simulink model "main_simulation"  (R2021a)
settings: Solver=VariableStepAuto  StartTime=0.0  StopTime=0.5  FixedStep=1e-4  RelTol=1e-6
settings Model: Creator=Federico  LastModifiedBy=Federico

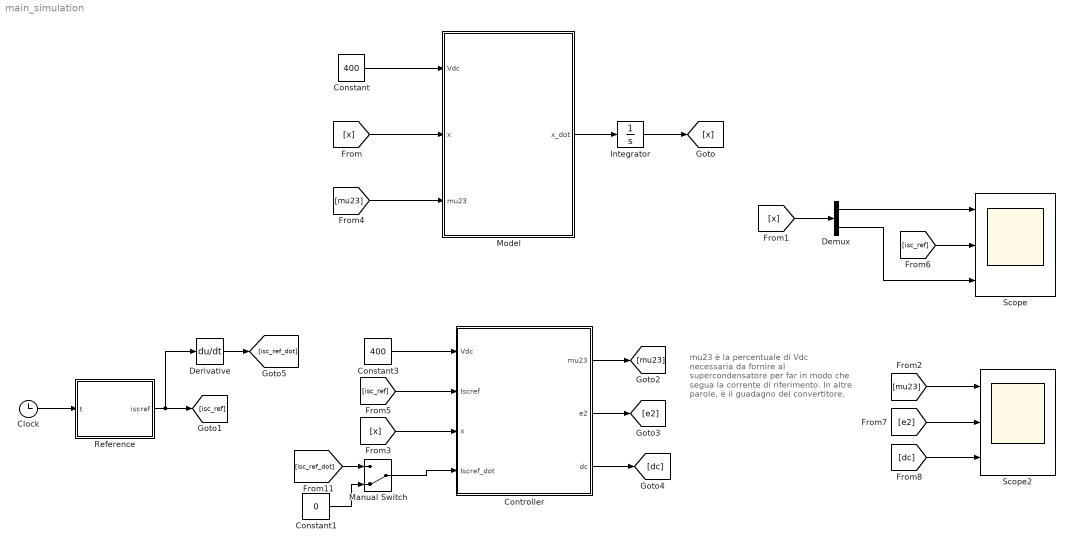
== system main_simulation ==
  note: mu23 è la percentuale di Vdc necessaria da fornire al supercondensatore per far in modo che segua la corrente di riferimento.
      | In altre parole, è il guadagno del convertitore.
  Clock : Clock
  Constant : Constant  Value=400
  Constant1 : Constant  Value=0
  Constant3 : Constant  Value=400
  Controller : MATLAB Function  TreatAsAtomicUnit=on
  Demux : Demux  Outputs=2
  Derivative : Derivative
  Integrator : Integrator  InitialCondition=[0;290]
  Manual Switch : ManualSwitch  CurrentSetting=0
  Model : MATLAB Function  TreatAsAtomicUnit=on
  Reference : MATLAB Function  TreatAsAtomicUnit=on
  Scope : Scope  NumInputPorts=3
  Scope2 : Scope  NumInputPorts=3
  wires:
  Controller/2(e2) -> [e2]
  Demux/2 -> Scope/3
  [isc_ref] -> Controller/2(Iscref)
  Reference/1(iscref) -> Derivative/1, [isc_ref]
  [mu23] -> Scope2/1
  [isc_ref] -> Scope/2
  Demux/1 -> Scope/1
  Integrator/1 -> [x]
  Clock/1 -> Reference/1(t)
  Constant3/1 -> Controller/1(Vdc)
  [x] -> Model/2(x)
  [x] -> Demux/1
  Model/1(x_dot) -> Integrator/1
  [x] -> Controller/3(x)
  Controller/1(mu23) -> [mu23]
  [e2] -> Scope2/2
  Constant/1 -> Model/1(Vdc)
  Derivative/1 -> [isc_ref_dot]
  Controller/3(dc) -> [dc]
  [mu23] -> Model/3(mu23)
  [isc_ref_dot] -> Manual Switch/1
  Constant1/1 -> Manual Switch/2
  Manual Switch/1 -> Controller/4(Iscref_dot)
  [dc] -> Scope2/3

== matlab function main_simulation/Controller ==
  data: Vdc input; Iscref input; mu23 output; x input; e2 output; Iscref_dot input; dc output
function [mu23, e2, dc] = controller(Vdc,Iscref,x,Iscref_dot)

c2=1000;
R2 = 20;
L2 = 3.3;
%Iscref_dot = 0;
e2 = x(1)-Iscref;
mu23 = L2/Vdc*(c2*e2 + (x(2)-R2*x(1))/L2 - Iscref_dot);

dc = mu23/(1+mu23); %duty cycle nel buck boost converter
if dc>=1
    dc = 1;
end
if dc <=0
    dc = 0;
end

end

== matlab function main_simulation/Model ==
  data: Vdc input; x_dot output; x input; mu23 input
function x_dot = model(Vdc,x,mu23)
Rsc = 66; %mOhm
Csc = 21.27; %Faraday

R2 = 20;
L2 = 3.3;

%modello mediato sul periodo di switching:
isc_dot = -mu23*(Vdc/L2) - (R2/L2)*x(1) + x(2)/L2;
vsc_dot = (-1/(Rsc*Csc))*(x(2)+Rsc*x(1));

x_dot = [isc_dot; vsc_dot];

end

== matlab function main_simulation/Reference ==
  data: t input; iscref output
function iscref = fcn(t)

iscref=0;
if t<=0.15
    iscref = 10;
end
if (t>0.15 && t<= 0.30)
    iscref = -20;
end
if (t>0.30)
    iscref = 5;
end

end
